simulink library "lib_parallel_comp"  (Simulink 7.4)
settings: Solver=ode45  StartTime=0.0  StopTime=10.0  RelTol=1e-3
values from neighbouring files (symbols this model uses):
  P_D = x(1)    [get_tank_deriv.m]
  Ts = 0.05    [const_sim.m]    (also in cost_functions.m; read_cpu_times.m; read_cpu_times_serial.m)
  uoff1 = [0.304, 0.405, 1, 0]'    [const_sim.m]
  uoff2 = [0.304, -1, 0.393, 0]'    [const_sim.m]
undefined symbols (not defined in the file or in its folder): n_delay
libraries: lib_compressor x2, dspsrcs4 x1
settings Model: Creator=chkajon  LastModifiedBy=chkajon

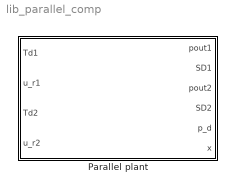
== system lib_parallel_comp ==
  Parallel plant : Subsystem  mask{disturbances_on=off, disturbances_symm=off, dist_t_in=0, dist1_in=0, dist2_in=0}
      mask prompts: disturbances_on "Activate disturbances"; disturbances_symm "Symmetric disturbances"; dist_t_in "Disturbance times (up to 2)"; dist1_in "Disturbance 1 values (u1in, u1out, ud[, u2in, u2out])"; dist2_in "Disturbance 2 values"
      mask init:
      | dist1 = zeros(5,1);
      | dist2 = dist1;
      | dist_t = zeros(2,1);
      | 
      | if disturbances_on
      |     for i=1:min(5,length(dist1_in))
      |         dist1(i) = dist1_in(i);
      |     end
      |     for i=1:min(5,length(dist2_in))
      |         dist2(i) = dist2_in(i);
      |     end
      |     for i=1:min(2,length(dist_t_in))
      |         dist_t(i) = dist_t_in(i);
      |     end
      |     
      |     if disturbances_symm
      |         dist1(4) = dist1(1);
      |         dist1(5) = dist1(2);
      |         dist2(4) = dist2(1);
      |         dist2(5) = dist2(2);
      |     end
      | end

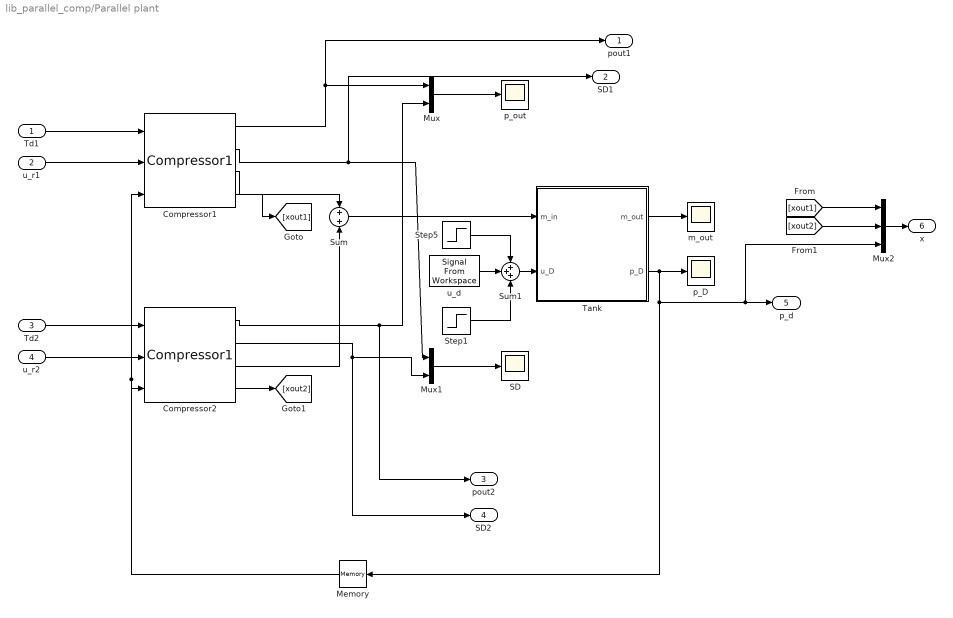
== system lib_parallel_comp/Parallel plant ==
  Td1 : Inport  OutDataType=fixdt(1, 16)  OutScaling=2^0
  u_r1 : Inport  Port=2  OutDataType=fixdt(1, 16)  OutScaling=2^0
  Td2 : Inport  Port=3  OutDataType=fixdt(1, 16)  OutScaling=2^0
  u_r2 : Inport  Port=4  OutDataType=fixdt(1, 16)  OutScaling=2^0
  Compressor1 : lib_compressor/Compressor1  SystemSampleTime=-1  Td_off=uoff1(1)  u_in=uoff1(2)  u_out=uoff1(3)  u_rec=uoff1(4)  t_delay=n_delay(2)*Ts  use_dist=on  u_out_dist=[dist1(1); dist2(1)]  u_out_time=dist_t  u_in_dist=[dist1(2); dist2(2)]  u_in_time=dist_t
  Compressor2 : lib_compressor/Compressor1  SystemSampleTime=-1  Td_off=uoff2(1)  u_in=uoff2(2)  u_out=uoff2(3)  u_rec=uoff2(4)  t_delay=n_delay(2)*Ts  use_dist=on  u_out_dist=[dist1(4); dist2(4)]  u_out_time=dist_t  u_in_dist=[dist1(5); dist2(5)]  u_in_time=dist_t
  Memory : Memory  X0=P_D
  Mux : Mux  Inputs=2
  Mux1 : Mux  Inputs=2
  Mux2 : Mux  Inputs=3
  SD : Scope
      settings: YMin=-2.5  YMax=0
  Step1 : Step  Time=dist_t(2)  After=dist2(3)  SampleTime=0
  Step5 : Step  Time=dist_t(1)  After=dist1(3)  SampleTime=0
  Sum : Sum  OutDataType=fixdt(1, 16)  OutScaling=2^0
  Sum1 : Sum  Inputs=+++  OutDataType=fixdt(1, 16)  OutScaling=2^0
  Tank : Subsystem
  m_out : Scope
      settings: SaveName=ScopeData2
  p_D : Scope
      settings: YMin=1.01  YMax=1.075  SaveName=ScopeData3
  p_out : Scope
  u_d : dspsrcs4/Signal From Workspace  SystemSampleTime=-1  X=u_d  Ts=Ts  nsamps=1  OutputAfterFinalValue=Holding final value  ignoreOrWarnInputAndFrameLengths=off
  pout1 : Outport  OutDataType=fixdt(1, 16)  OutScaling=2^0
  SD1 : Outport  Port=2  OutDataType=fixdt(1, 16)  OutScaling=2^0
  pout2 : Outport  Port=3  OutDataType=fixdt(1, 16)  OutScaling=2^0
  SD2 : Outport  Port=4  OutDataType=fixdt(1, 16)  OutScaling=2^0
  p_d : Outport  Port=5  OutDataType=fixdt(1, 16)  OutScaling=2^0
  x : Outport  Port=6  OutDataType=fixdt(1, 16)  OutScaling=2^0
  wires:
  Compressor1/3 -> Sum/1
  Tank/1(m_out) -> m_out/1
  Tank/2(p_D) -> p_D/1, p_d/1, Mux2/3, Memory/1
  Compressor1/1 -> Mux/1, pout1/1
  Compressor1/2 -> Mux1/1, SD1/1
  Compressor2/1 -> Mux/2, pout2/1
  Compressor2/2 -> Mux1/2, SD2/1
  Td1/1 -> Compressor1/1
  u_r1/1 -> Compressor1/2
  Sum/1 -> Tank/1(m_in)
  Mux1/1 -> SD/1
  Mux/1 -> p_out/1
  Td2/1 -> Compressor2/1
  u_r2/1 -> Compressor2/2
  Memory/1 -> Compressor1/3, Compressor2/3
  Compressor2/3 -> Sum/2
  [xout1] -> Mux2/1
  Compressor1/4 -> [xout1]
  Compressor2/4 -> [xout2]
  [xout2] -> Mux2/2
  Mux2/1 -> x/1
  Sum1/1 -> Tank/2(u_D)
  Step5/1 -> Sum1/1
  u_d/1 -> Sum1/2
  Step1/1 -> Sum1/3

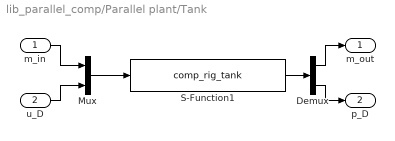
== system lib_parallel_comp/Parallel plant/Tank ==
  m_in : Inport  OutDataType=fixdt(1, 16)  OutScaling=2^0
  u_D : Inport  Port=2  OutDataType=fixdt(1, 16)  OutScaling=2^0
  Demux : Demux  Outputs=2
  Mux : Mux  Inputs=2
  S-Function1 : S-Function  FunctionName=comp_rig_tank  Parameters=[], P_D  EnableBusSupport=off
  m_out : Outport  OutDataType=fixdt(1, 16)  OutScaling=2^0
  p_D : Outport  Port=2  OutDataType=fixdt(1, 16)  OutScaling=2^0
  wires:
  S-Function1/1 -> Demux/1
  Demux/1 -> m_out/1
  Demux/2 -> p_D/1
  Mux/1 -> S-Function1/1
  m_in/1 -> Mux/1
  u_D/1 -> Mux/2
